simulink model "disturbance_visualization_reduced"  (R2016b)
settings: Solver=VariableStepAuto  StartTime=0.0  StopTime=10.0  RelTol=1e-3
values from neighbouring files (symbols this model uses):
  period = total_length/v    (= 0.0214401685393)    [disturbance_visualization_constants.m]    (also in run_air_spring_disturbed_connected_slx.m = 0.142401119403)
  slot_depth = -0.0127    [disturbance_visualization_constants.m]    (also in run_air_spring_disturbed_connected_slx.m)
  track_drift_incremental = 0.001016    [disturbance_input_2.m]    (also in disturbance_input_3.m; disturbance_visualization_constants.m; run_air_spring_disturbed_connected_slx.m)
  track_drift_max = 0.01016    [disturbance_input_2.m]    (also in disturbance_input_3.m; disturbance_visualization_constants.m; run_air_spring_disturbed_connected_slx.m)
  wth_pulse_phase_delay = track_length/v    (= 0.021404494382)    [disturbance_visualization_constants.m]    (also in run_air_spring_disturbed_connected_slx.m = 0.142164179104)
  wth_pulse_width = 100*slot_length/total_length    (= 0.166389351082)    [disturbance_visualization_constants.m]    (also in run_air_spring_disturbed_connected_slx.m)
undefined symbols (not defined in the file or in its folder): DiscIntNeverNeededParam
settings Model: Creator=Jared  LastModifiedBy=Jared

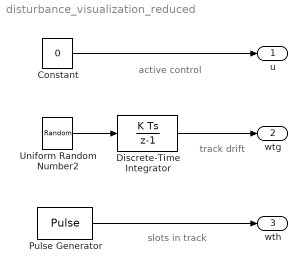
== system disturbance_visualization_reduced ==
  note: active control
  note: slots in track
  note: track drift
  Constant : Constant  Value=0
  Discrete-Time Integrator : DiscreteIntegrator  InitialConditionSetting=State (most efficient)  SampleTime=-1  LimitOutput=on  UpperSaturationLimit=track_drift_max  LowerSaturationLimit=-track_drift_max  ICPrevOutput=DiscIntNeverNeededParam  ICPrevScaledInput=DiscIntNeverNeededParam
  Pulse Generator : DiscretePulseGenerator  PulseType=Time based  Amplitude=slot_depth  Period=period  PulseWidth=wth_pulse_width  PhaseDelay=wth_pulse_phase_delay
  Uniform Random Number2 : UniformRandomNumber  Minimum=-track_drift_incremental  Maximum=track_drift_incremental  SampleTime=period
  u : Outport
  wtg : Outport  Port=2
  wth : Outport  Port=3
  wires:
  Pulse Generator/1 -> wth/1
  Discrete-Time Integrator/1 -> wtg/1
  Uniform Random Number2/1 -> Discrete-Time Integrator/1
  Constant/1 -> u/1
